simulink model "Astatic_DigitalPolynomial"  (R2021a)
settings: Solver=FixedStepAuto  StartTime=0.0  StopTime=STime  FixedStep=1e-3  RelTol=1e-6
undefined symbols (not defined in the file): C, C_polya, J, Kp, Mc, new_c, new_d, new_n, new_r, r0a, R_polya, Ra, Ta, Tp, TPert
settings Model: Creator=akangmufti  LastModifiedBy=akangmufti

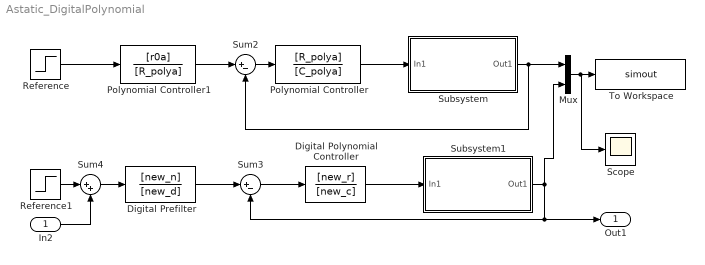
== system Astatic_DigitalPolynomial ==
  In2 : Inport
  Digital Polynomial Controller : DiscreteFilter  Numerator=[new_r]  Denominator=[new_c]  SampleTime=1e-3
  Digital Prefilter : DiscreteFilter  Numerator=[new_n]  Denominator=[new_d]  SampleTime=1e-3
  Mux : Mux  Inputs=2
  Polynomial Controller : TransferFcn  Numerator=[R_polya]  Denominator=[C_polya]
  Polynomial Controller1 : TransferFcn  Numerator=[r0a]  Denominator=[R_polya]
  Reference : Step  Time=1e-3  SampleTime=0
  Reference1 : Step  Time=1e-3  SampleTime=0
  Scope : Scope
  Subsystem : Subsystem
  Subsystem1 : Subsystem
  Sum2 : Sum  Inputs=|+-
  Sum3 : Sum  Inputs=|+-
  Sum4 : Sum  Inputs=|++
  To Workspace : ToWorkspace  VariableName=simout  SampleTime=-1
  Out1 : Outport
  wires:
  Subsystem/1(Out1) -> Mux/1, Sum2/2
  Sum2/1 -> Polynomial Controller/1
  Reference/1 -> Polynomial Controller1/1
  Polynomial Controller1/1 -> Sum2/1
  Mux/1 -> Scope/1, To Workspace/1
  Polynomial Controller/1 -> Subsystem/1(In1)
  Digital Polynomial Controller/1 -> Subsystem1/1(In1)
  Sum3/1 -> Digital Polynomial Controller/1
  Sum4/1 -> Digital Prefilter/1
  Digital Prefilter/1 -> Sum3/1
  In2/1 -> Sum4/2
  Reference1/1 -> Sum4/1
  Subsystem1/1(Out1) -> Mux/2, Sum3/2, Out1/1

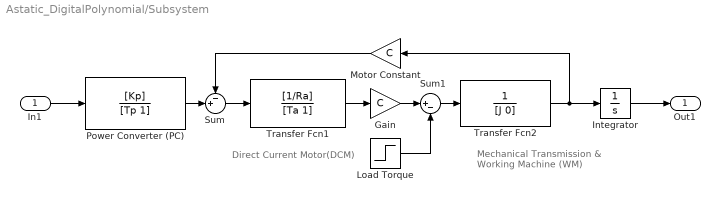
== system Astatic_DigitalPolynomial/Subsystem ==
  note: Direct Current Motor(DCM)
  note: Mechanical Transmission &
      | Working Machine (WM)
  In1 : Inport
  Gain : Gain  Gain=C
  Integrator : Integrator  ContinuousStateAttributes='AngularPosition'
  Load Torque : Step  Time=TPert  After=Mc  SampleTime=0
  Motor Constant : Gain  Gain=C
  Power Converter (PC) : TransferFcn  Numerator=[Kp]  Denominator=[Tp 1]
  Sum : Sum  Inputs=-+|
  Sum1 : Sum  Inputs=|+-
  Transfer Fcn1 : TransferFcn  Numerator=[1/Ra]  Denominator=[Ta 1]  ContinuousStateAttributes='Current'
  Transfer Fcn2 : TransferFcn  Denominator=[J 0]  ContinuousStateAttributes='Omega'
  Out1 : Outport
  wires:
  Transfer Fcn2/1 -> Integrator/1, Motor Constant/1
  Power Converter (PC)/1 -> Sum/2
  Gain/1 -> Sum1/1
  Sum1/1 -> Transfer Fcn2/1
  Sum/1 -> Transfer Fcn1/1
  Transfer Fcn1/1 -> Gain/1
  Motor Constant/1 -> Sum/1
  In1/1 -> Power Converter (PC)/1
  Load Torque/1 -> Sum1/2
  Integrator/1 -> Out1/1

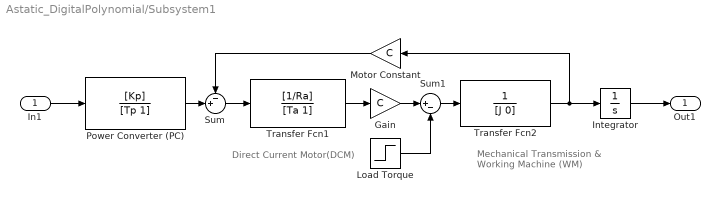
== system Astatic_DigitalPolynomial/Subsystem1 ==
  note: Mechanical Transmission &
      | Working Machine (WM)
  note: Direct Current Motor(DCM)
  In1 : Inport
  Gain : Gain  Gain=C
  Integrator : Integrator  ContinuousStateAttributes='AngularPosition'
  Load Torque : Step  Time=TPert  After=Mc  SampleTime=0
  Motor Constant : Gain  Gain=C
  Power Converter (PC) : TransferFcn  Numerator=[Kp]  Denominator=[Tp 1]
  Sum : Sum  Inputs=-+|
  Sum1 : Sum  Inputs=|+-
  Transfer Fcn1 : TransferFcn  Numerator=[1/Ra]  Denominator=[Ta 1]  ContinuousStateAttributes='Current'
  Transfer Fcn2 : TransferFcn  Denominator=[J 0]  ContinuousStateAttributes='Omega'
  Out1 : Outport
  wires:
  Integrator/1 -> Out1/1
  Load Torque/1 -> Sum1/2
  In1/1 -> Power Converter (PC)/1
  Motor Constant/1 -> Sum/1
  Transfer Fcn1/1 -> Gain/1
  Sum/1 -> Transfer Fcn1/1
  Sum1/1 -> Transfer Fcn2/1
  Gain/1 -> Sum1/1
  Power Converter (PC)/1 -> Sum/2
  Transfer Fcn2/1 -> Motor Constant/1, Integrator/1
